simulink model "Adaptive_Cruise_Control_System"  (R2016b)
settings: Solver=FixedStepAuto  StartTime=0.0  StopTime=110.0  RelTol=1e-3
libraries: simulink x5, autolibshared x2
(part 3 of 3)

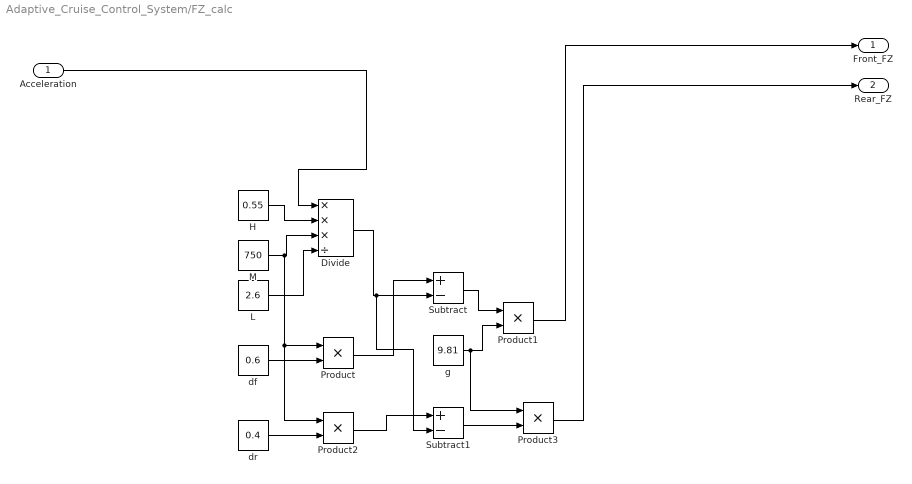
== system Adaptive_Cruise_Control_System/FZ_calc ==
  Acceleration : Inport
  Divide : Product  Inputs=***/
  H : Constant  Value=0.55
  L : Constant  Value=2.6
  M : Constant  Value=750
  Product{,1..3} (4 alike) : Product
  Subtract : Sum  Inputs=+-
  Subtract1 : Sum  Inputs=+-
  df : Constant  Value=0.6
  dr : Constant  Value=0.4
  g : Constant  Value=9.81
  Front_FZ : Outport
  Rear_FZ : Outport  Port=2
  wires:
  L/1 -> Divide/4
  M/1 -> Product2/1, Product/1, Divide/3
  Product/1 -> Subtract/1
  Divide/1 -> Subtract1/2, Subtract/2
  df/1 -> Product/2
  Subtract/1 -> Product1/1
  Acceleration/1 -> Divide/1
  H/1 -> Divide/2
  Product3/1 -> Rear_FZ/1
  Product1/1 -> Front_FZ/1
  Subtract1/1 -> Product3/2
  g/1 -> Product3/1, Product1/2
  dr/1 -> Product2/2
  Product2/1 -> Subtract1/1
